simulink model "ADRC_ang_acc_change"  (R2020b)
settings: Solver=VariableStepAuto  StartTime=0.0  StopTime=10.0  RelTol=1e-3
undefined symbols (not defined in the file): b, b0, g, g1, g2, kd, kd1, ki1, kp, kp1, V, wo
libraries: pid_lib x1
settings Model: Creator=11814  LastModifiedBy=11814
settings DataIOCC: ReturnWorkspaceOutputs=off
settings DebuggingCC: ArithmeticOperatorsInVariantConditions=warning
settings SFSimCC: SimUseLocalCustomCode=off  CustomCodeUndefinedFunction=UseInterfaceOnly
settings RTWCC: RTWUseLocalCustomCode=off
settings CodeAppCC: StateflowObjectComments=on

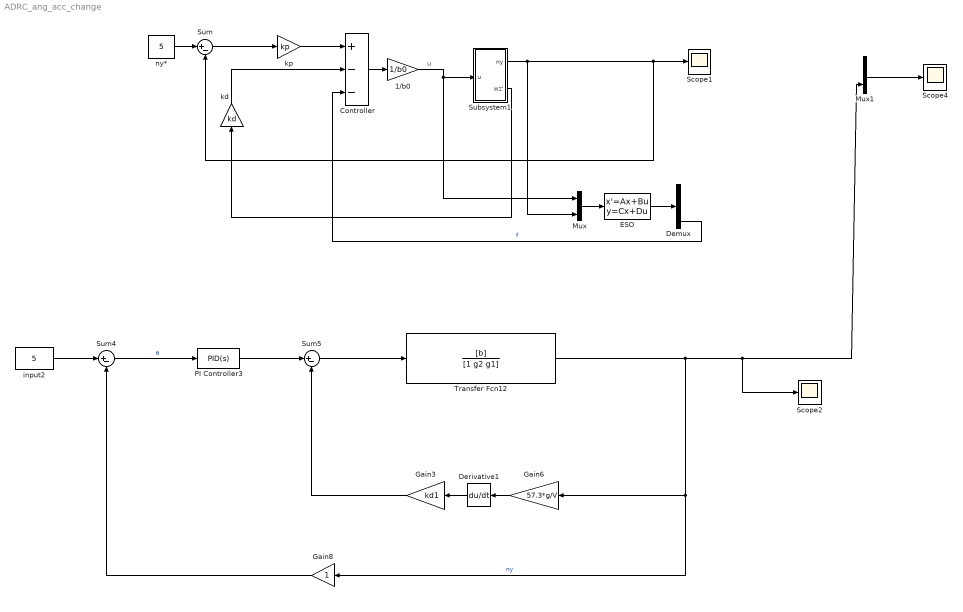
== system ADRC_ang_acc_change ==
  note: u
  1/b0 : Gain  Gain=1/b0
  Controller : Sum  Inputs=+--
  Demux : Demux  Outputs=3
  Derivative1 : Derivative
  ESO : StateSpace  A=[-3*wo 1 0; -3*wo^2 0 1; -wo^3 0 0]  B=[0 3*wo; b0 3*wo^2; 0 wo^3]  C=eye(3)  D=[0 0; 0 0; 0 0]  InitialCondition=0
  Gain3 : Gain  Gain=kd1
  Gain6 : Gain  Gain=57.3*g/V
  Gain8 : Gain
  Mux : Mux  Inputs=2
  Mux1 : Mux  Inputs=2
  PI Controller3 : pid_lib/PID Controller  Controller=PID  Form=Parallel  TimeDomain=Continuous-time  UseExternalTs=off  SampleTime=-1  IntegratorMethod=Forward Euler  FilterMethod=Forward Euler  ControllerParametersSource=internal  P=kp1  I=ki1  D=0  UseFilter=on  N=100  TunerSelectOption=Transfer Function Based (PID Tuner App)  InitialConditionSource=internal  InitialConditionForIntegrator=0  InitialConditionForFilter=0  DifferentiatorICPrevScaledInput=0  ExternalReset=none  TrackingMode=off  Kt=1  LimitOutput=off  SatLimitsSource=internal  UpperSaturationLimit=inf  LowerSaturationLimit=-inf  LinearizeAsGain=on  AntiWindupMode=none  Kb=1  POutMin=[]  POutMax=[]  IOutMin=[]  IOutMax=[]  DOutMin=[]  DOutMax=[]  NOutMin=[]  NOutMax=[]  SumOutMin=[]  SumOutMax=[]  SaturationOutMin=[]  SaturationOutMax=[]  PParamMin=[]  PParamMax=[]  IParamMin=[]  IParamMax=[]  DParamMin=[]  DParamMax=[]  NParamMin=[]  NParamMax=[]  KbParamMin=[]  KbParamMax=[]  KtParamMin=[]  KtParamMax=[]  KbOutMin=[]  KbOutMax=[]  KtOutMin=[]  KtOutMax=[]  IntegratorOutMin=[]  IntegratorOutMax=[]  FilterOutMin=[]  FilterOutMax=[]  SumI1OutMin=[]  SumI1OutMax=[]  SumI2OutMin=[]  SumI2OutMax=[]  SumI3OutMin=[]  SumI3OutMax=[]  SumI4OutMin=[]  SumI4OutMax=[]  SumDOutMin=[]  SumDOutMax=[]  DifferentiatorOutMin=[]  DifferentiatorOutMax=[]  FilterDiffOutCoefMin=[]  FilterDiffOutCoefMax=[]  ReciprocalOutMin=[]  ReciprocalOutMax=[]  SumDenOutMin=[]  SumDenOutMax=[]  SumNumOutMin=[]  SumNumOutMax=[]  DivideOutMin=[]  DivideOutMax=[]  UdiffTsProdOutMin=[]  UdiffTsProdOutMax=[]  NTsProdOutMin=[]  NTsProdOutMax=[]  UintegralTsProdOutMin=[]  UintegralTsProdOutMax=[]  UngainTsProdOutMin=[]  UngainTsProdOutMax=[]  IntegratorContinuousStateAttributes=''  IntegratorStateMustResolveToSignalObject=off  IntegratorRTWStateStorageClass=Auto  FilterContinuousStateAttributes=''  FilterStateMustResolveToSignalObject=off  FilterRTWStateStorageClass=Auto  ParallelPVariant=InternalParameters  IdealPVariant=Disabled  IVariant=InternalParameters  DVariant=InternalParameters  IntegratorVariant=Continuous  SatVariant=Disabled  AWVariant=Passthrough  PCopyVariant=Disabled  TRVariant=Disabled  FdbkBlocksVariant=Forward  IdealPFdbkVariant=Disabled  SatFdbkVariant=Disabled  DerivativeFilterVariant=ContFilter  NVariant=InternalParameters  NCopyVariant=Disabled  FilterICVariant=InternalICsFilter  IntegratorICVariant=InternalICs  ExternalResetVariant=Disabled  TRSumVariant=Passthrough  SumFdbkVariant=Disabled  SumVariant=Sum_PID  TsampFilterVariant=InternalTs  TsampNgainVariant=Passthrough  TsampIntegralVariant=Passthrough  ExternalSaturationOutDataTypeStr=Inherit: Same as second input
  Scope1 : Scope
  Scope2 : Scope
  Scope4 : Scope
  Subsystem1 : Subsystem
  Sum : Sum  Inputs=|+-
  Sum4 : Sum  Inputs=|+-
  Sum5 : Sum  Inputs=|+-
  Transfer Fcn12 : TransferFcn  Numerator=[b]  Denominator=[1 g2 g1]
  input2 : Constant  Value=5
  kd : Gain  Gain=kd
  kp : Gain  Gain=kp
  ny* : Constant  Value=5
  wires:
  Mux/1 -> ESO/1
  Subsystem1/1(ny) -> Mux/2, Scope1/1, Sum/2
  Demux/3 -> Controller/3  "f"
  kd/1 -> Controller/2
  Sum/1 -> kp/1
  kp/1 -> Controller/1
  ESO/1 -> Demux/1
  ny*/1 -> Sum/1
  Controller/1 -> 1/b0/1
  1/b0/1 -> Mux/1, Subsystem1/1(u)
  Subsystem1/2(wz') -> kd/1
  PI Controller3/1 -> Sum5/1
  Gain8/1 -> Sum4/2
  Derivative1/1 -> Gain3/1
  Gain3/1 -> Sum5/2
  input2/1 -> Sum4/1
  Transfer Fcn12/1 -> Scope2/1, Mux1/2, Gain8/1, Gain6/1  "ny"
  Gain6/1 -> Derivative1/1
  Sum5/1 -> Transfer Fcn12/1
  Sum4/1 -> PI Controller3/1  "e"
  Mux1/1 -> Scope4/1

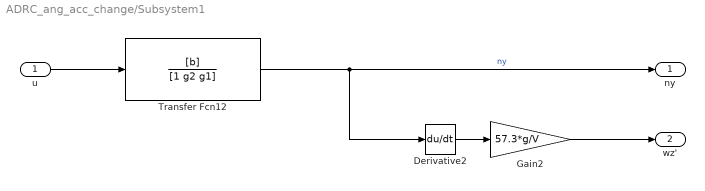
== system ADRC_ang_acc_change/Subsystem1 ==
  u : Inport
  Derivative2 : Derivative
  Gain2 : Gain  Gain=57.3*g/V
  Transfer Fcn12 : TransferFcn  Numerator=[b]  Denominator=[1 g2 g1]
  ny : Outport
  wz' : Outport  Port=2
  wires:
  u/1 -> Transfer Fcn12/1
  Transfer Fcn12/1 -> Derivative2/1, ny/1  "ny"
  Derivative2/1 -> Gain2/1
  Gain2/1 -> wz'/1
